simulink model "sim_all_2019b"  (R2019b)
settings: Solver=VariableStepAuto  StartTime=0.0  StopTime=2000  RelTol=1e-3
undefined symbols (not defined in the file or in its folder): a1, a2, alpha1, alpha2, cornerA, cornerB, cornerC, cornerD, ctrl_clockwise, ctrl_int_bound_or, ctrl_int_bound_pos, ctrl_k_or, ctrl_k_pos, ctrl_Ki_vel, ctrl_Kp_v_pos, ctrl_Kp_vel, ctrl_TAM, ctrl_Ts, ctrl_va_uncontrolled, ctrl_vel_uncontrolled, D, dead_zone_limit, depth, DiscIntNeverNeededParam, distanceFromWall, initInspectedSide, initPoint, mod_A, mod_Cd_F, mod_Cd_M, mod_eta_init, mod_g, mod_h0, mod_Ixx, mod_Iyy, mod_Izz, mod_Kp_dot, mod_lat0, mod_lon0, mod_m, mod_Mq_dot, mod_ni_init, mod_Nr_dot, mod_p1, mod_p2, mod_p3, mod_p4, mod_p5, mod_p6, mod_R, mod_Rm, mod_t1, mod_t2, mod_t3, mod_t4, mod_t5, mod_t6, mod_W, mod_Xu_dot, mod_Yv_dot ... (+53)
libraries: simulink x8, cstblocks x6, simulink_extras x1
(part 3 of 6)

== system sim_all_2019b/Mission_supervisor_v3/Mission_Supervisor/Orientazione in profondità ==
  Pos_s : Inport
  Orp_s : Inport  Port=2
  Punto_iniz_patt : Inport  Port=3
  error_flag : Inport  Port=4
  Action Port : ActionPort  ActionPortLabel=case [ 104 ]:
  Constant{,1..3,6} (5 alike) : Constant  Value=nan
  MATLAB Function : MATLAB Function  TreatAsAtomicUnit=on  SystemSampleTime=Ts_supervisor
  Mux : Mux  Inputs=6
  Mux1 : Mux  Inputs=3
  delta_current_or_prof : Outport
  delta_stato_or_prof : Outport  Port=2
  Outport : Outport  Port=3
  wires:
  MATLAB Function/1(delta_current_or_prof) -> delta_current_or_prof/1
  MATLAB Function/2(delta_stato_or_prof) -> delta_stato_or_prof/1
  MATLAB Function/3(Pos_d) -> Mux/1
  Mux/1 -> Outport/1
  Constant1/1 -> Mux/3
  MATLAB Function/4(Dpp_d) -> Mux/4
  MATLAB Function/5(Orp_d) -> Mux/6
  Constant/1 -> Mux1/1
  Constant2/1 -> Mux1/2
  Constant6/1 -> Mux1/3
  Mux1/1 -> Mux/2
  Constant3/1 -> Mux/5
  Pos_s/1 -> MATLAB Function/1(Pos_s)
  Orp_s/1 -> MATLAB Function/2(Orp_s)
  Punto_iniz_patt/1 -> MATLAB Function/3(punto_iniz_patt)
  error_flag/1 -> MATLAB Function/4(error_flag)

== system sim_all_2019b/Mission_supervisor_v3/Mission_Supervisor/Orientazione in superficie ==
  Or_in : Inport
  error_flag : Inport  Port=2
  punto_iniz_patt : Inport  Port=3
  Pos_s : Inport  Port=4
  Or_s : Inport  Port=5
  Action Port : ActionPort  ActionPortLabel=case [ 302 ]:
  Constant{1..2,4..5} (4 alike) : Constant  Value=nan
  MATLAB Function : MATLAB Function  TreatAsAtomicUnit=on  SystemSampleTime=Ts_supervisor
  Mux : Mux  Inputs=6
  delta_current_or_sup : Outport
  delta_stato_or_sup : Outport  Port=2
  Outport : Outport  Port=3
  wires:
  Mux/1 -> Outport/1
  Constant1/1 -> Mux/3
  Constant4/1 -> Mux/5
  Or_in/1 -> MATLAB Function/1(Or_in)
  error_flag/1 -> MATLAB Function/2(error_flag)
  punto_iniz_patt/1 -> MATLAB Function/3(punto_iniz_patt)
  MATLAB Function/1(delta_current_or_sup) -> delta_current_or_sup/1
  MATLAB Function/2(delta_stato_or_sup) -> delta_stato_or_sup/1
  MATLAB Function/4(Or_d) -> Mux/2
  MATLAB Function/3(Pos_d) -> Mux/1
  Constant2/1 -> Mux/4
  Constant5/1 -> Mux/6
  Pos_s/1 -> MATLAB Function/4(Pos_s)
  Or_s/1 -> MATLAB Function/5(Or_s)

== system sim_all_2019b/Mission_supervisor_v3/Mission_Supervisor/Pattugliamento ==
  parete : Inport
  contatore : Inport  Port=2
  Pos_s : Inport  Port=3
  Dpp_s : Inport  Port=4
  Dps_s : Inport  Port=5
  Orp_s : Inport  Port=6
  Vel_s : Inport  Port=7
  error_flag : Inport  Port=8
  giro : Inport  Port=9
  Action Port : ActionPort  ActionPortLabel=case [ 201 ]:
  Constant{,1..2,6} (4 alike) : Constant  Value=nan
  MATLAB Function : MATLAB Function  TreatAsAtomicUnit=on  SystemSampleTime=Ts_supervisor
  Mux : Mux  Inputs=6
  Mux1 : Mux  Inputs=3
  delta_current_patt : Outport
  delta_stato_patt : Outport  Port=2
  Outport : Outport  Port=3
  wires:
  MATLAB Function/1(delta_current_patt) -> delta_current_patt/1
  MATLAB Function/2(delta_stato_patt) -> delta_stato_patt/1
  parete/1 -> MATLAB Function/1(parete)
  contatore/1 -> MATLAB Function/2(contatore)
  MATLAB Function/3(Pos_d) -> Mux/1
  Mux/1 -> Outport/1
  Mux1/1 -> Mux/2
  MATLAB Function/4(Vel_d) -> Mux/3
  MATLAB Function/5(Dpp_d) -> Mux/4
  Constant/1 -> Mux1/1
  Constant2/1 -> Mux1/2
  Constant6/1 -> Mux1/3
  Pos_s/1 -> MATLAB Function/3(Pos_s)
  Dpp_s/1 -> MATLAB Function/4(Dpp_s)
  Dps_s/1 -> MATLAB Function/5(Dps_s)
  Vel_s/1 -> MATLAB Function/7(Vel_s)
  Orp_s/1 -> MATLAB Function/6(Orp_s)
  error_flag/1 -> MATLAB Function/8(error_flag)
  giro/1 -> MATLAB Function/9(giro)
  Constant1/1 -> Mux/5
  MATLAB Function/6(Orp_d) -> Mux/6

== system sim_all_2019b/Mission_supervisor_v3/Mission_Supervisor/Posizionamento ==
  Pos_s : Inport
  Or_s : Inport  Port=2
  punto iniziale : Inport  Port=3
  Or_in : Inport  Port=4
  error_flag : Inport  Port=5
  Action Port : ActionPort  ActionPortLabel=case [ 102 ]:
  Constant{,1..3} (4 alike) : Constant  Value=nan
  MATLAB Function : MATLAB Function  TreatAsAtomicUnit=on  SystemSampleTime=Ts_supervisor
  Mux : Mux  Inputs=6
  delta_current_posiz : Outport
  delta_stato_posiz : Outport  Port=2
  Outport : Outport  Port=3
  wires:
  MATLAB Function/1(delta_current_posiz) -> delta_current_posiz/1
  MATLAB Function/2(delta_stato_posiz) -> delta_stato_posiz/1
  MATLAB Function/3(Pos_d) -> Mux/1
  MATLAB Function/4(Or_d) -> Mux/2
  Mux/1 -> Outport/1
  Constant/1 -> Mux/3
  Constant1/1 -> Mux/6
  Constant2/1 -> Mux/5
  Pos_s/1 -> MATLAB Function/1(Pos_s)
  punto iniziale/1 -> MATLAB Function/3(punto_iniziale)
  Or_in/1 -> MATLAB Function/4(Or_in)
  Or_s/1 -> MATLAB Function/2(Or_s)
  error_flag/1 -> MATLAB Function/5(error_flag)
  Constant3/1 -> Mux/4

== system sim_all_2019b/Mission_supervisor_v3/Mission_Supervisor/Rientro ==
  Pos_s : Inport
  Or_in : Inport  Port=2
  error_flag : Inport  Port=3
  Dps_s : Inport  Port=4
  Dpp_s : Inport  Port=5
  Or_s : Inport  Port=6
  Action Port : ActionPort  ActionPortLabel=case [ 303 ]:
  Constant{1..4} (4 alike) : Constant  Value=nan
  MATLAB Function : MATLAB Function  TreatAsAtomicUnit=on  SystemSampleTime=Ts_supervisor
  Mux : Mux  Inputs=6
  delta_current_rient : Outport
  delta_stato_rient : Outport  Port=2
  Outport : Outport  Port=3
  wires:
  MATLAB Function/1(delta_current_rient) -> delta_current_rient/1
  MATLAB Function/2(delta_stato_rient) -> delta_stato_rient/1
  MATLAB Function/3(Pos_d) -> Mux/1
  Mux/1 -> Outport/1
  Constant1/1 -> Mux/3
  Constant2/1 -> Mux/4
  Constant3/1 -> Mux/5
  Constant4/1 -> Mux/6
  Pos_s/1 -> MATLAB Function/1(Pos_s)
  MATLAB Function/4(Or_d) -> Mux/2
  Or_in/1 -> MATLAB Function/2(Or_in)
  error_flag/1 -> MATLAB Function/3(error_flag)
  Dps_s/1 -> MATLAB Function/4(Dps_s)
  Dpp_s/1 -> MATLAB Function/5(Dpp_s)
  Or_s/1 -> MATLAB Function/6(Or_s)

== system sim_all_2019b/Mission_supervisor_v3/Mission_Supervisor/Risalita ==
  delta_SOS : Inport
  Pos_s : Inport  Port=2
  Dpp_s : Inport  Port=3
  Orp_s : Inport  Port=4
  Dps_s : Inport  Port=5
  Dps_fin : Inport  Port=6
  error_flag : Inport  Port=7
  SOS_205 : Inport  Port=8
  Action Port : ActionPort  ActionPortLabel=case [ 301 ]:
  Constant{,1,3,6} (4 alike) : Constant  Value=nan
  MATLAB Function : MATLAB Function  TreatAsAtomicUnit=on  SystemSampleTime=Ts_supervisor
  Mux : Mux  Inputs=6
  Mux1 : Mux  Inputs=3
  delta_current_ris : Outport
  delta_stato_ris : Outport  Port=2
  Outport : Outport  Port=3
  wires:
  MATLAB Function/1(delta_current_ris) -> delta_current_ris/1
  MATLAB Function/2(delta_stato_ris) -> delta_stato_ris/1
  MATLAB Function/3(Pos_d) -> Mux/1
  Mux/1 -> Outport/1
  Mux1/1 -> Mux/2
  Constant1/1 -> Mux/3
  MATLAB Function/4(Dpp_d) -> Mux/4
  Constant/1 -> Mux1/1
  Constant3/1 -> Mux1/2
  Constant6/1 -> Mux1/3
  MATLAB Function/5(Dps_d) -> Mux/5
  Pos_s/1 -> MATLAB Function/2(Pos_s)
  Dpp_s/1 -> MATLAB Function/3(Dpp_s)
  MATLAB Function/6(Orp_d) -> Mux/6
  delta_SOS/1 -> MATLAB Function/1(delta_SOS)
  Orp_s/1 -> MATLAB Function/4(Orp_s)
  Dps_s/1 -> MATLAB Function/5(Dps_s)
  Dps_fin/1 -> MATLAB Function/6(Dps_fin)
  error_flag/1 -> MATLAB Function/7(error_flag)
  SOS_205/1 -> MATLAB Function/8(SOS_205)

== system sim_all_2019b/Model/Vehicle Model/P1 ==
  note: n is the rotational speed of the thruster
      | V is the speed component of the water along the thruster axis
      |
      | n is saturated according to data
      | a dead zone is considered according to data
      | the thruster is characterised by 1st order dynamics (tau = 0.2s)
  n1 [rad/s] : Inport
  V1 [m/s] : Inport  Port=2
  Dead Zone : DeadZone  LowerValue=-dead_zone_limit  UpperValue=dead_zone_limit  SaturateOnIntegerOverflow=on
  Propeller1 : MATLAB Function  TreatAsAtomicUnit=on
  Saturation : Saturate  UpperLimit=n_max  LowerLimit=-n_max
  Transfer Fcn : TransferFcn  Denominator=[0.2 1]
  T1 : Outport
  wires:
  V1 [m/s]/1 -> Propeller1/2(V1)
  Saturation/1 -> Propeller1/1(n1)
  Transfer Fcn/1 -> Saturation/1
  Dead Zone/1 -> Transfer Fcn/1
  n1 [rad/s]/1 -> Dead Zone/1
  Propeller1/1(T1) -> T1/1

== system sim_all_2019b/Model/Vehicle Model/P2 ==
  note: n is the rotational speed of the thruster
      | V is the speed component of the water along the thruster axis
      |
      | n is saturated according to data
      | a dead zone is considered according to data
      | the thruster is characterised by 1st order dynamics (tau = 0.2s)
  n2 [rad/s] : Inport
  V2 [m/s] : Inport  Port=2
  Dead Zone : DeadZone  LowerValue=-dead_zone_limit  UpperValue=dead_zone_limit  SaturateOnIntegerOverflow=on
  Propeller2 : MATLAB Function  TreatAsAtomicUnit=on
  Saturation : Saturate  UpperLimit=n_max  LowerLimit=-n_max
  Transfer Fcn : TransferFcn  Denominator=[0.2 1]
  T2 : Outport
  wires:
  V2 [m/s]/1 -> Propeller2/2(V2)
  Saturation/1 -> Propeller2/1(n2)
  Transfer Fcn/1 -> Saturation/1
  Dead Zone/1 -> Transfer Fcn/1
  n2 [rad/s]/1 -> Dead Zone/1
  Propeller2/1(T2) -> T2/1

== system sim_all_2019b/Model/Vehicle Model/P3 ==
  note: n is the rotational speed of the thruster
      | V is the speed component of the water along the thruster axis
      |
      | n is saturated according to data
      | a dead zone is considered according to data
      | the thruster is characterised by 1st order dynamics (tau = 0.2s)
  n3 [rad/s] : Inport
  V3 [m/s] : Inport  Port=2
  Dead Zone : DeadZone  LowerValue=-dead_zone_limit  UpperValue=dead_zone_limit  SaturateOnIntegerOverflow=on
  Propeller3 : MATLAB Function  TreatAsAtomicUnit=on
  Saturation : Saturate  UpperLimit=n_max  LowerLimit=-n_max
  Transfer Fcn : TransferFcn  Denominator=[0.2 1]
  T3 : Outport
  wires:
  V3 [m/s]/1 -> Propeller3/2(V3)
  Saturation/1 -> Propeller3/1(n3)
  Transfer Fcn/1 -> Saturation/1
  Dead Zone/1 -> Transfer Fcn/1
  n3 [rad/s]/1 -> Dead Zone/1
  Propeller3/1(T3) -> T3/1

== system sim_all_2019b/Model/Vehicle Model/P4 ==
  note: n is the rotational speed of the thruster
      | V is the speed component of the water along the thruster axis
      |
      | n is saturated according to data
      | a dead zone is considered according to data
      | the thruster is characterised by 1st order dynamics (tau = 0.2s)
  n4 [rad/s] : Inport
  V4 [m/s] : Inport  Port=2
  Dead Zone : DeadZone  LowerValue=-dead_zone_limit  UpperValue=dead_zone_limit  SaturateOnIntegerOverflow=on
  Propeller4 : MATLAB Function  TreatAsAtomicUnit=on
  Saturation : Saturate  UpperLimit=n_max  LowerLimit=-n_max
  Transfer Fcn : TransferFcn  Denominator=[0.2 1]
  T4 : Outport
  wires:
  V4 [m/s]/1 -> Propeller4/2(V4)
  Saturation/1 -> Propeller4/1(n4)
  Transfer Fcn/1 -> Saturation/1
  Dead Zone/1 -> Transfer Fcn/1
  n4 [rad/s]/1 -> Dead Zone/1
  Propeller4/1(T4) -> T4/1

== system sim_all_2019b/Model/Vehicle Model/P5 ==
  note: n is the rotational speed of the thruster
      | V is the speed component of the water along the thruster axis
      |
      | n is saturated according to data
      | a dead zone is considered according to data
      | the thruster is characterised by 1st order dynamics (tau = 0.2s)
  n5 [rad/s] : Inport
  V5 [m/s] : Inport  Port=2
  Dead Zone : DeadZone  LowerValue=-dead_zone_limit  UpperValue=dead_zone_limit  SaturateOnIntegerOverflow=on
  Propeller5 : MATLAB Function  TreatAsAtomicUnit=on
  Saturation : Saturate  UpperLimit=n_max  LowerLimit=-n_max
  Transfer Fcn : TransferFcn  Denominator=[0.2 1]
  T5 : Outport
  wires:
  V5 [m/s]/1 -> Propeller5/2(V5)
  Saturation/1 -> Propeller5/1(n5)
  Transfer Fcn/1 -> Saturation/1
  Dead Zone/1 -> Transfer Fcn/1
  n5 [rad/s]/1 -> Dead Zone/1
  Propeller5/1(T5) -> T5/1

== system sim_all_2019b/Model/Vehicle Model/P6 ==
  note: n is the rotational speed of the thruster
      | V is the speed component of the water along the thruster axis
      |
      | n is saturated according to data
      | a dead zone is considered according to data
      | the thruster is characterised by 1st order dynamics (tau = 0.2s)
  n6 [rad/s] : Inport
  V6 [m/s] : Inport  Port=2
  Dead Zone : DeadZone  LowerValue=-dead_zone_limit  UpperValue=dead_zone_limit  SaturateOnIntegerOverflow=on
  Propeller6 : MATLAB Function  TreatAsAtomicUnit=on
  Saturation : Saturate  UpperLimit=n_max  LowerLimit=-n_max
  Transfer Fcn : TransferFcn  Denominator=[0.2 1]
  T6 : Outport
  wires:
  V6 [m/s]/1 -> Propeller6/2(V6)
  Saturation/1 -> Propeller6/1(n6)
  Transfer Fcn/1 -> Saturation/1
  Dead Zone/1 -> Transfer Fcn/1
  n6 [rad/s]/1 -> Dead Zone/1
  Propeller6/1(T6) -> T6/1

== system sim_all_2019b/Navigation/Extended Kalman Filter/AHRS__check ==
  AHRS_new : Inport
  MATLAB Function4 : MATLAB Function  TreatAsAtomicUnit=on
  Memory4 : Memory
  flag_AHRS : Outport
  AHRS_now : Outport  Port=2
  wires:
  AHRS_new/1 -> MATLAB Function4/1(AHRS_new)
  Memory4/1 -> MATLAB Function4/2(AHRS_old)
  MATLAB Function4/1(flag_AHRS) -> flag_AHRS/1
  MATLAB Function4/2(AHRS_now) -> Memory4/1, AHRS_now/1

== system sim_all_2019b/Navigation/Extended Kalman Filter/CORREZIONE ==
  x_k|k-1 : Inport
  P_k|k-1 : Inport  Port=2
  e : Inport  Port=3
  H : Inport  Port=4
  R : Inport  Port=5
  nav_flag_init : Inport  Port=6
  MATLAB Function : MATLAB Function  TreatAsAtomicUnit=on  SystemSampleTime=nav_DT
  x_k|k : Outport
  P_k|k : Outport  Port=2
  wires:
  x_k|k-1/1 -> MATLAB Function/1(x_k_k_1)
  P_k|k-1/1 -> MATLAB Function/2(P_k_k_1)
  e/1 -> MATLAB Function/3(e)
  H/1 -> MATLAB Function/4(H)
  MATLAB Function/1(x_k) -> x_k|k/1
  MATLAB Function/2(P_k) -> P_k|k/1
  nav_flag_init/1 -> MATLAB Function/6(nav_flag_init)
  R/1 -> MATLAB Function/5(R_k)

== system sim_all_2019b/Navigation/Extended Kalman Filter/DVL_check ==
  DVL_new : Inport
  MATLAB Function4 : MATLAB Function  TreatAsAtomicUnit=on
  Memory4 : Memory
  flag_DVL : Outport
  DVL_now : Outport  Port=2
  wires:
  DVL_new/1 -> MATLAB Function4/1(DVL_new)
  Memory4/1 -> MATLAB Function4/2(DVL_old)
  MATLAB Function4/1(flag_DVL) -> flag_DVL/1
  MATLAB Function4/2(DVL_now) -> Memory4/1, DVL_now/1

== system sim_all_2019b/Navigation/Extended Kalman Filter/MISURA VIRTUALE ==
  x_k|k-1 : Inport
  flag_vect : Inport  Port=2
  mis_vect : Inport  Port=3
  J : Inport  Port=4
  MATLAB Function : MATLAB Function  TreatAsAtomicUnit=on  SystemSampleTime=nav_DT
  e : Outport
  H : Outport  Port=2
  wires:
  x_k|k-1/1 -> MATLAB Function/1(x_k_k_1)
  mis_vect/1 -> MATLAB Function/3(mis_vect)
  flag_vect/1 -> MATLAB Function/2(flag_vect)
  MATLAB Function/1(e) -> e/1
  MATLAB Function/2(H) -> H/1
  J/1 -> MATLAB Function/4(J)

== system sim_all_2019b/Navigation/Extended Kalman Filter/PREDIZIONE ==
  x0 : Inport
  P0 : Inport  Port=2
  x_k-1|k-1 : Inport  Port=3
  u_k-1 : Inport  Port=4
  P_k-1|k-1 : Inport  Port=5
  J : Inport  Port=6
  L : Inport  Port=7
  Q_k-1 : Inport  Port=8
  nav_flag_init : Inport  Port=9
  Passo di Predizione : MATLAB Function  TreatAsAtomicUnit=on  SystemSampleTime=nav_DT
  x_k|k-1 : Outport
  P_k|k-1 : Outport  Port=2
  flag_init : Outport  Port=3
  wires:
  Passo di Predizione/1(x_k) -> x_k|k-1/1
  Passo di Predizione/2(P_k) -> P_k|k-1/1
  u_k-1/1 -> Passo di Predizione/4(u_k_1)
  x_k-1|k-1/1 -> Passo di Predizione/3(x_k_1)
  P_k-1|k-1/1 -> Passo di Predizione/5(P_k_1)
  J/1 -> Passo di Predizione/6(J)
  Q_k-1/1 -> Passo di Predizione/8(Q_k_1)
  P0/1 -> Passo di Predizione/2(P0)
  x0/1 -> Passo di Predizione/1(x0)
  L/1 -> Passo di Predizione/7(L)
  nav_flag_init/1 -> Passo di Predizione/9("nav_flag_init ")
  Passo di Predizione/3(nav_flag_init) -> flag_init/1

== system sim_all_2019b/Navigation/Extended Kalman Filter/Q_error ==
  flag_AHRS : Inport
  flag_DVL : Inport  Port=2
  Q : Inport  Port=3
  MATLAB Function4 : MATLAB Function  TreatAsAtomicUnit=on
  Memory : Memory
  Q_k : Outport
  wires:
  MATLAB Function4/1(Q_k) -> Q_k/1, Memory/1
  flag_AHRS/1 -> MATLAB Function4/3(flag_AHRS)
  flag_DVL/1 -> MATLAB Function4/4(flag_DVL)
  Memory/1 -> MATLAB Function4/2(Q_k_1)
  Q/1 -> MATLAB Function4/1(Q)

== system sim_all_2019b/Sensors/BLOCCO GYRO1/Subsystem ==
  t : Inport  SampleTime=sens_Sample_time_GYRO
  GEOD to NED : MATLAB Function  TreatAsAtomicUnit=on
  Bias_G : Outport
  wires:
  t/1 -> GEOD to NED/1(t)
  GEOD to NED/1(Bias_G) -> Bias_G/1

== matlab function sim_all_2019b/Mission_supervisor_v3/Mission_Supervisor/MATLAB Function1 ==
  data: punto_iniz_patt output size=3; initInspectedSide parameter; distanceFromWall parameter; initPoint parameter; Or_in output; dps_fin output; cornerA parameter; cornerB parameter; cornerC parameter; cornerD parameter; relativeDirection parameter; alfa output
function [punto_iniz_patt, Or_in, dps_fin, alfa] = ambiente(initInspectedSide,distanceFromWall,initPoint,cornerA, cornerB, cornerC, cornerD, relativeDirection)
 
    %% Unità di misura 
    
    % punto_iniz_patt, initPoint, cornerA, cornerB, cornerC, cornerD        [deg, deg, m]
    % Or_in                                                                 [rad, rad, rad]
    % dps_fin,distanceFromWall                                              [m]
    % alfa                                                                  [rad]
    % relativeDirection                                                     [deg]

    %% Inizializzazione variabili
    
    % Valori dati da file relativi agli angoli del bacino
    iP = initPoint;
    A = cornerA;
    B = cornerB;
    C = cornerC;
    D = cornerD;

    coder.extrinsic('evalin', 'wgs84Ellipsoid', 'geodetic2ned');
    coder.extrinsic('evalin', 'wgs84Ellipsoid', 'ned2geodetic');

    % Inizializzazione di alcune variabili
    xA = 0; yA = 0; zA = 0; xB = 0; yB = 0; zB = 0; xC = 0; yC = 0; zC = 0; 
    xD = 0; yD = 0; zD = 0; xiP = 0; yiP = 0; ziP = 0;
    xpipAB = 0; ypipAB = 0; zpipAB = 0; xpipBC = 0; ypipBC = 0; zpipBC = 0; 
    xpipCD = 0; ypipCD = 0; zpipCD = 0; xpipDA = 0; ypipDA = 0; zpipDA = 0;
    depth_in = initPoint(3);
    Or_in = [0; 0; 0];
    
    % Conversione da Geodetic a NED delle posizioni degli angoli e del punto iniziale
    wgs84 = wgs84Ellipsoid; % Per il corretto funzionamento e' necessario installare un 
                            % pacchetto aggiuntivo in Matlab qualora non fosse presente
    [xA, yA, zA] = geodetic2ned(A(1), A(2), 0, C(1), C(2), 0, wgs84);
    [xB, yB, zB] = geodetic2ned(B(1), B(2), 0, C(1), C(2), 0, wgs84);
    [xC, yC, zC] = geodetic2ned(C(1), C(2), 0, C(1), C(2), 0, wgs84);
    [xD, yD, zD] = geodetic2ned(D(1), D(2), 0, C(1), C(2), 0, wgs84);
    [xiP, yiP, ziP] = geodetic2ned(iP(1), iP(2), 0, C(1), C(2), 0, wgs84);
    inizio = [xiP; yiP; depth_in];

    % Punti centrali delle pareti
    pcAB = [(xB + xA)/2; (yB + yA)/2; depth_in];
    pcBC = [(xB + xC)/2; (yB + yC)/2; depth_in];   
    pcCD = [(xC + xD)/2;(yC + yD)/2; depth_in];
    pcDA = [(xD + xA)/2; (yD + yA)/2; depth_in];

    % Lunghezze delle pareti
    AB = sqrt((xA - xB)^2 + (yA - yB)^2); 
    BC = sqrt((xB - xC)^2 + (yB - yC)^2); 
    CD = sqrt((xC - xD)^2 + (yC - yD)^2); 
    DA = sqrt((xD - xA)^2 + (yD - yA)^2); 
    
    dW = distanceFromWall;

    %% Calcolo punto di inizio pattugliamento a meta' parete

    % Calcolo degli angoli relativi tra le pareti 
    thetaBC = acos(yB/BC);          
    thetaCD = acos(yD/CD);
    gammaAB = acos((yB - yA)/AB);
    thetaAB = pi - gammaAB;
    gammaDA = acos((yA - yD)/DA);

    % Punti di inizio pattugliamento a seconda di quale parete è scelta come
    % parete iniziale
    
    dbpc = sqrt((pcAB(1) - xB)^2 + (pcAB(2) - yB)^2);
    hpb = sqrt(dbpc^2 + dW^2);
    alfa1 = - acos(dbpc/hpb);
    gammaab = pi - (gammaAB + alfa1);
    pcab1 = [hpb * sin(gammaab), hpb * cos(gammaab)];
    pipAB = [xB + pcab1(1); yB + pcab1(2); depth_in];

    dcpc = sqrt(pcBC(1)^2 + pcBC(2)^2);
    hpc = sqrt(dcpc^2 + dW^2);
    alfabc = acos(dcpc/hpc);
    gammaBC = thetaBC + alfabc;
    pipBC = [hpc * sin(gammaBC); hpc * cos(gammaBC); depth_in];

    dcdpc = sqrt(pcCD(1)^2 + pcCD(2)^2);
    hpcd = sqrt(dcdpc^2 + dW^2);
    alfacd = acos(dcdpc/hpcd);
    gammaCD = thetaCD - alfacd;
    pipCD = [hpcd * sin(gammaCD); hpcd * cos(gammaCD); depth_in];

    dapc = sqrt((pcDA(1) - xA)^2 + (pcDA(2) - yA)^2);
    hpda = sqrt(dapc^2 + dW^2);
    alfada = acos(dapc/hpda);
    gammada = pi + (gammaDA + alfada);
    pcda1 = [hpda * sin(gammada), hpda * cos(gammada)];
    pipDA = [xA + pcda1(1); yA + pcda1(2); depth_in];
    
    % Si convertono i punti "pip" da NED a Geodetic 
    [xpipAB, ypipAB, zpipAB] = ned2geodetic(pipAB(1), pipAB(2), pipAB(3), C(1), C(2), 0, wgs84);
    [xpipBC, ypipBC, zpipBC] = ned2geodetic(pipBC(1), pipBC(2), pipBC(3), C(1), C(2), 0, wgs84);
    [xpipCD, ypipCD, zpipCD] = ned2geodetic(pipCD(1), pipCD(2), pipCD(3), C(1), C(2), 0, wgs84);
    [xpipDA, ypipDA, zpipDA] = ned2geodetic(pipDA(1), pipDA(2), pipDA(3), C(1), C(2), 0, wgs84);

    pipAB_geodetic = [xpipAB; ypipAB; depth_in];
    pipBC_geodetic = [xpipBC; ypipBC; depth_in];
    pipCD_geodetic = [xpipCD; ypipCD; depth_in];
    pipDA_geodetic = [xpipDA; ypipDA; depth_in];

    %% Calcolo angolo di orientazione iniziale in direzione del punto di inizio  pattugliamento (rispetto al nord)

    % Versore orinetato verso il nord n = [1, 0, 0];
    
    % Vettori che vanno dal punto di partenza al punto di inizio pattugliamento
    
    iAB = pipAB - inizio;
    iBC = pipBC - inizio;
    iCD = pipCD - inizio;
    iDA = pipDA - inizio;

    % Angoli tra direzione Nord e il vettore che porta verso il punto di inizio pattugliamento. 
    % Sono gli angoli di orientazione iniziale desiderata. 
    theta1 = atan2d(iAB(2),iAB(1));
    theta2 = atan2d(iBC(2),iBC(1));
    theta3 = atan2d(iCD(2),iCD(1));
    theta4 = atan2d(iDA(2),iDA(1));
    
    % Si raccoglie in un vettore
    theta = [deg2rad(theta1), deg2rad(theta2), deg2rad(theta3), deg2rad(theta4)];

    %% Si calcolano gli angoli interni dei vertici
    
    alfaC = thetaCD - thetaBC;
    alfaB = pi - (thetaAB-thetaBC);
    alfaA = thetaAB - gammaDA;
    alfaD = 2*pi - alfaA - alfaB - alfaC;
    alfa = [alfaA; alfaB; alfaC; alfaD];    %Utilizzati poi in fase di manovra

    %% Calcolo distanza dalla parete successiva a partire da meta'  parete

    % Sono le distanze da metà parete alla parete successiva
    dABpc = sqrt((pcAB(1) - xB)^2 + (pcAB(2) - yB)^2);
    dBCpc = sqrt(pcBC(1)^2 + pcBC(2)^2);
    dCDpc = sqrt(pcCD(1)^2 + pcCD(2)^2);
    dDApc = sqrt((pcDA(1) - xA)^2 + (pcDA(2) - yA)^2);


    %% Scelta delle condizioni

    % In base al valore di parete iniziale si assegnano i giusti valori per i 
    % riferimenti da utilizzare nei vari stati
    
    if initInspectedSide == 1

        punto_iniz_patt = pipAB_geodetic;
        Or_in = [0; 0; theta(1)];
        dps_fin = dABpc;

    elseif initInspectedSide == 2

        punto_iniz_patt = pipBC_geodetic;
        Or_in = [0; 0; theta(2)];
        dps_fin = dBCpc;

    elseif initInspectedSide == 3

        punto_iniz_patt = pipCD_geodetic;
        Or_in = [0; 0; theta(3)];
        dps_fin = dCDpc;

    else

        punto_iniz_patt = pipDA_geodetic;
        Or_in = [0; 0; theta(4)];
        dps_fin = dDApc;

    end
                                                                            %****TEST*****%
                                                                            %Or_in = [1; 1; 1];

end

== matlab function sim_all_2019b/Controller_mk4_v3/C_pos/C_pos_Y ==
  data: err_int output; pos input; vel output; k input; ctrl_vel_uncontrolled parameter; ctrl_int_bound_pos parameter
%% Azione proporzionale
function [err_int, vel] = fcn(pos, k, ctrl_vel_uncontrolled, ctrl_int_bound_pos)
    v = 0;
    err_int = 0;
    vel_des = ctrl_vel_uncontrolled;    % velocità impostata se 'lontani'
    brake_dist = 1/k*vel_des;           % distanza di frenata
    if pos >= brake_dist                % se ho spazio per frenare mantengo la velocità
        v = vel_des;
    end
    if pos <= -brake_dist               % lontani in direzione negativa
        v = -vel_des;
    end
    if  abs(pos) < brake_dist           % se è vicino il proporzionale gestisce la frenata
        v = k*pos;
    end
    vel = v;
    if abs(pos) < ctrl_int_bound_pos    % per il regime può essere utile una azione integrale
        err_int = pos;                  % err_int va ad un integratore
    end

== matlab function sim_all_2019b/Mission_supervisor_v3/Mission_Supervisor/Inizio/MATLAB Function ==
  data: current_state output; parete_attuale output; stato_interno output; Pos_d output size=3; Pos_s input; error_flag input; attesa input; initInspectedSide parameter; initPoint parameter; timer parameter; SOS parameter
function [current_state, parete_attuale, stato_interno, Pos_d] =  Inizio(Pos_s, error_flag, attesa, initInspectedSide, initPoint, timer, SOS)
    
    disp("Inizio");
    
    %% Unita' di misura
    
    % Pos_d, Pos_s, initPoint                                                [deg, deg, m]
    % attesa, timer                                                          [s]
    
    %% Inizializzazione variabili
    
    % Mantenimento di stato_interno al valore
    % desiderato durante la permanenza del sistema nello stato corrente.
    stato_interno = 100;

    % Se non si ricevono dati dal GPS per un tempo superiore ad una soglia
    % massima di attesa, la missione viene interrotta poiché non è
    % possibile localizzarsi nel bacino
    if ((isnan(Pos_s(1)) || isnan(Pos_s(2))) && (attesa > timer))
        SOS = 1;
        disp("EMERGENZA: mancata ricezione dati da GPS");
    end
    
    %% Preparazione dei riferimenti 
    
        % Parete di inizio pattugliamento
        parete_attuale = initInspectedSide;
        
        % Posizione di inizio missione
        Pos_d = initPoint; 
        
        
    %% Transizione di stato effettiva
    
        % Quando i riferimenti sono correttamente settati
        % viene comunicato agli altri moduli il passaggio di stato
        current_state = 100;  
        
    %% Decisione dello stato successivo
    
     if error_flag == 1
        disp("EMERGENZA: errore segnalato dagli altri sottosistemi");
        SOS = 1;
     end
    
    % Si verifica lo stato di emergenza e la ricezione di misure dal GPS
    if (SOS == 0 && ((isnan(Pos_s(1)) == false && isnan(Pos_s(2)) == false))) 
        
        stato_interno = 101;   % Si passa allo stato successivo
    else
        if SOS == 1
           
            stato_interno = 304; % Politica di emergenza: si passa in fine missione   
        end
    end

end

== matlab function sim_all_2019b/Mission_supervisor_v3/Mission_Supervisor/MATLAB Function ==
  data: parete_iniziale input; verso input; parete output; contatore input; initInspectedSide parameter; current_state input; giro output
function [parete, giro] = aggiorna_parete(parete_iniziale, verso, contatore, initInspectedSide,current_state)
   
 %% Corpo funzione 
    
    % A seconda del senso di pattugliamento si ha l'aggiornamento del valore
    % di parete attuale. 
    
    if(strcmp(verso,'clockwise') == 1)
        giro = 0;
        parete = mod((parete_iniziale + contatore),4);
        if(parete == 0)
            parete = 4;
        end
    else % 'counterclockwise'
        giro = 1;
        parete = parete_iniziale - contatore;
        if(parete <= 0)
            parete = parete+4;
        end
    end

    % Per stati precedenti al 201, si forza questa variabile a
    % mantenere il valore pari al valore iniziale. 
    if(current_state < 201)
        parete = initInspectedSide;
    end
    
end

== matlab function sim_all_2019b/Mission_supervisor_v3/Mission_Supervisor/Orientazione Iniziale/MATLAB Function ==
  data: delta_stato_or_iniz output; delta_current_or_iniz output; Pos_d output size=3; Pos_s input size=3; Or_s input size=3; Or_in input; initPoint parameter size=3; Or_d output size=3; error_flag input; soglia_or parameter; soglia_SOS_pos parameter; SOS parameter; soglia_SOS_or parameter
function [delta_stato_or_iniz, delta_current_or_iniz, Pos_d, Or_d] = Orientazione_iniziale(Pos_s, Or_s, Or_in, initPoint, error_flag, soglia_or, soglia_SOS_pos, SOS, soglia_SOS_or)

    disp("Orientazione iniziale");
    
    %% Unità di misura 
    
    % Pos_d, Pos_s, initPoint, soglia_SOS_pos                                [deg, deg, m]
    % Or_d, Or_s, Or_in, soglia_or, soglia_SOS_or                            [rad, rad, rad]
    
    %% Inizializzazione variabili
    
    % Mantenimento dello stato_interno al valore
    % desiderato durante la permanenza del sistema nello stato corrente.
    delta_stato_or_iniz = 0;
    
    % Variabile utilizzata per segnalare il momento in cui
    % effettuare la transizione di stato. 
    pronti = false;
    
    %% Preparazione dei riferimenti da fornire ai blocchi successivi
                
    % Posizione da mantenere
    Pos_d = initPoint; 
   
    % Orientazione desiderata per raggiungere
    % il punto di inizio pattugliamento
    Or_d = Or_in;
    
    % Quando i riferimenti sono correttamente settati
    % il passaggio di stato viene comunicato agli altri moduli
    delta_current_or_iniz = 101 - 100;
    
    
    %% Verifiche
    
    % Si verifica il mantenimento della posizione 
    % e la ricezione della stima di orientazione
    if (abs(Pos_s(1) - Pos_d(1)) > soglia_SOS_pos(1) || ...
        abs(Pos_s(2) - Pos_d(2)) > soglia_SOS_pos(2) || ...
        abs(Pos_s(3) - Pos_d(3)) > soglia_SOS_pos(3) || ...
        isnan(Or_s(1)) || isnan(Or_s(2)) || isnan(Or_s(3)) || ...
        abs(Or_s(1) - Or_d(1)) > soglia_SOS_or(1) || ...
        abs(Or_s(2) - Or_d(2)) > soglia_SOS_or(2))
    
        SOS = 1;
        disp("EMERGENZA:");
        
        if (abs(Pos_s(1) - Pos_d(1)) > soglia_SOS_pos(1))
            disp("Rilevato errore sulla posizione X");
        end
        if (abs(Pos_s(2) - Pos_d(2)) > soglia_SOS_pos(2))
            disp("Rilevato errore sulla posizione Y");
        end
        if (abs(Pos_s(3) - Pos_d(3)) > soglia_SOS_pos(3))
            disp("Rilevato errore sulla profondita Z");
        end
        if (isnan(Or_s(1)))
            disp("Mancata ricezione della prima componente di orientazione");
        end
        if (isnan(Or_s(2)))
            disp("Mancata ricezione della seconda componente di orientazione");
        end
        if (isnan(Or_s(3)))
            disp("Mancata ricezione della terza componente di orientazione");
        end
        if (abs(Or_s(1) - Or_d(1)) > soglia_SOS_or(1))
            disp("Rilevato errore sulla rotazione di roll");
        end
        if (abs(Or_s(2) - Or_d(2)) > soglia_SOS_or(2))
            disp("Rilevato errore sulla rotazione di pitch");
        end
    end

    if error_flag == 1
        disp("EMERGENZA: errore segnalato dagli altri sottosistemi");
        SOS = 1;
    end
    
    % Si verifica di aver raggiunto l'orientazione desiderata
    if (SOS == 0 && ...
        (abs(Or_s(3) - Or_d(3)) < soglia_or(3)))
    
        pronti = true;
        
    end
       
    %% Decisione dello stato successivo
    
    if pronti == true
        
        delta_stato_or_iniz = 102 - 101; % Transizione eseguita correttamente
    end
        
    if SOS == 1
            
            delta_stato_or_iniz = 304 - 101; % Transizione nello stato di emergenza
    end
    % Si rimane nello stato corrente

end

== matlab function sim_all_2019b/Mission_supervisor_v3/Mission_Supervisor/Immersione/MATLAB Function ==
  data: soglia_pos parameter; delta_current_immers output; delta_stato_immers output; Pos_d output size=3; Or_d output size=3; Pos_s input; depth parameter; punto_iniz_patt input; Or_in input; error_flag input; soglia_SOS_pos parameter; SOS parameter
function [delta_current_immers, delta_stato_immers, Pos_d, Or_d]=Immersione(soglia_pos, Pos_s, depth, punto_iniz_patt, Or_in, error_flag, soglia_SOS_pos, SOS)

    disp("Immersione");
    
    %% Unità di misura 
    
    % Pos_d, Pos_s, punto_iniz_patt, soglia_pos, soglia_SOS_pos            [deg, deg, m]
    % Or_d, Or_in                                                          [rad, rad, rad]
    % distanceFromWall, depth                                              [m]


    %% Inizializzazione variabili
    
    % Utilizzata durante la permanenza nello stato corrente
    delta_stato_immers = 0;
    
    pronti = false; 
    
    %% Preparazione dei riferimenti da fornire ai blocchi successivi
    
    % Posizione da raggiungere
    Pos_d = [punto_iniz_patt(1); punto_iniz_patt(2); depth];
                                                                            %*****TEST******%
                                                                            %Pos_d = [43; 11; 0];
    
    % Orientazione da mantenere
    Or_d = Or_in;
    
    % Transizione di stato effettiva
    delta_current_immers = 103 - 102;  
        
       
    %% Verifiche
    
    % Verifica della corretta posizione
    if (abs(Pos_s(1) - Pos_d(1)) > soglia_SOS_pos(1) || ...
        abs(Pos_s(2) - Pos_d(2)) > soglia_SOS_pos(2))
    
        SOS = 1;
        disp("EMERGENZA:"); 
        
        if (abs(Pos_s(1) - Pos_d(1)) > soglia_SOS_pos(1))
            disp("Rilevato errore sulla posizione X");
        end
        
        if (abs(Pos_s(2) - Pos_d(2)) > soglia_SOS_pos(2))
            disp("Rilevato errore sulla posizione Y");
        end

    end
    
    if error_flag == 1
        disp("EMERGENZA: errore segnalato dagli altri sottosistemi");
        SOS = 1;
    end
    
    % Si verifica di aver raggiunto la profondità desiderata 
    if (SOS == 0 && ...
        abs(Pos_s(3) - Pos_d(3)) < soglia_pos(3))
    
        pronti = true;
    end
    
    
    %% Decisione dello stato successivo
    
    if pronti == true
        
        delta_stato_immers = 104 - 103; % Transizione eseguita correttamente
    end 
    if SOS == 1
            
            delta_stato_immers = 301 - 103; % Transizione nello stato di emergenza
    end
    % Si rimane nello stato corrente

end

== matlab function sim_all_2019b/Mission_supervisor_v3/Mission_Supervisor/Orientazione in profondità/MATLAB Function ==
  data: delta_current_or_prof output; delta_stato_or_prof output; Pos_d output size=3; Dpp_d output; Orp_d output; Pos_s input; Orp_s input; relativeDirection parameter; depth parameter; punto_iniz_patt input; error_flag input; soglia_orp parameter; soglia_SOS_pos parameter; SOS parameter; distanceFromWall parameter
function [delta_current_or_prof, delta_stato_or_prof, Pos_d, Dpp_d, Orp_d] = Orientazione_profondita(Pos_s, Orp_s, relativeDirection, depth, punto_iniz_patt, error_flag, soglia_orp, soglia_SOS_pos, SOS, distanceFromWall)

    disp("Orientazione in profondita");
    
    %% Unità di misura 
    
    % Pos_d, Pos_s, punto_iniz_patt, soglia_SOS_pos                        [deg, deg, m]
    % Orp_d, Orp_s, soglia_orp                                             [rad]
    % relativeDirection                                                    [deg]
    % Dpp_d, depth, distanceFromWall                                       [m]

    %% Inizializzazione variabili
    
    % Utilizzata per la permanenza nello stato corrente
    delta_stato_or_prof = 0;
    
    pronti = false;

    %% Preparazione dei riferimenti da fornire ai blocchi successivi
                
    % Posizione da mantenere
    Pos_d = [punto_iniz_patt(1); punto_iniz_patt(2); depth];
                                                                            %*****TEST******%
                                                                            %Pos_d = [43; 11; 0];
    
  
    % Orientazione da raggiungere
    Orp_d = deg2rad(relativeDirection);
    
    % Distanza dalla parete da mantenere
    Dpp_d = distanceFromWall;
    
    
    % Transizione di stato effettiva
    delta_current_or_prof = 104 - 103; 
    
    
    %% Verifiche
    
    % Verifica della corretta posizione
    if (abs(Pos_s(1) - Pos_d(1)) > soglia_SOS_pos(1) || ...
        abs(Pos_s(2) - Pos_d(2)) > soglia_SOS_pos(2) || ...
        abs(Pos_s(3) - Pos_d(3)) > soglia_SOS_pos(3))
    
        SOS = 1;
        disp("EMERGENZA:");
        
        if (abs(Pos_s(1) - Pos_d(1)) > soglia_SOS_pos(1))
            disp("Rilevato errore sulla posizione X");
        end
        if (abs(Pos_s(2) - Pos_d(2)) > soglia_SOS_pos(2))
            disp("Rilevato errore sulla posizione Y");
        end
        if (abs(Pos_s(3) - Pos_d(3)) > soglia_SOS_pos(3))
            disp("Rilevato errore sulla profondita Z");
        end
        
    end
    
    if error_flag == 1
        disp("EMERGENZA: errore segnalato dagli altri sottosistemi");
        SOS = 1;
    end
     
    % Si verifica di aver raggiunto l'orientazione desiderata
    if (SOS == 0 && ...
        abs(Orp_s - Orp_d) < soglia_orp)
    
        pronti = true;
    end
    
    %% Decisione dello stato successivo
    
    if pronti == true
        
        delta_stato_or_prof = 201 - 104; % Transizione eseguita correttamente
    end
    if SOS == 1
            
            delta_stato_or_prof = 301 - 104; % Transizione nello stato di emergenza
    end
    
    % Si rimane nello stato corrente
    

end

== matlab function sim_all_2019b/Mission_supervisor_v3/Mission_Supervisor/Frenata pattugliamento/MATLAB Function ==
  data: delta_current_fren_patt output; delta_stato_fren_patt output; contatore input; Pos_d output size=3; Dpp_d output; Dps_d output; Orp_d output; Pos_s input; Dpp_s input; Dps_s input; Orp_s input; distanceFromWall parameter; relativeDirection parameter; depth parameter; error_flag input; soglia_SOS_orp parameter; soglia_SOS_pos parameter; soglia_SOS_parete parameter; SOS parameter; soglia_parete parameter
function [delta_current_fren_patt, delta_stato_fren_patt, Pos_d, Dpp_d, Dps_d, Orp_d] = Frenata_pattugliamento(contatore, Pos_s, Dpp_s, Dps_s, Orp_s, distanceFromWall, relativeDirection, depth, error_flag, soglia_SOS_orp, soglia_SOS_pos, soglia_SOS_parete, SOS,soglia_parete)

    disp("Frenata (durante il pattugliamento)");
    
    %% Unità di misura 
    
    % Pos_d, Pos_s, soglia_SOS_pos                                                                 [deg, deg, m]
    % Orp_d, Orp_s, soglia_SOS_orp                                                                 [rad]
    % relativeDirection                                                                            [deg]
    % Dpp_d, Dps_d, Dpp_s, Dps_s, distanceFromWall, depth, soglia_SOS_parete, soglia_parete        [m]

    %% Inizializzazione variabili
   
    % Utilizzata per permanere nello stato corrente
    delta_stato_fren_patt = contatore;
    
    pronti = false;
    
    %% Preparazione dei riferimenti da fornire ai blocchi successivi
    
    % Profondità da mantenere
    Pos_d = [nan; nan; depth];
                                                                            %*****TEST******%
                                                                            %Pos_d = [nan; nan; 0];
    
    % Distanza dalla parete da mantenere
    Dpp_d = distanceFromWall;
    Dps_d = distanceFromWall;
    
    % Orientazione da mantenere
    Orp_d = deg2rad(relativeDirection);
    
    % Transizione di stato effettiva
    delta_current_fren_patt = 202 - 201 + contatore;  
    
    
    %% Verifiche
    
    % Verifica sulla corretta orientazione, profondità e distanza dalla parete pattugliata
    if (abs(Orp_s - Orp_d) > soglia_SOS_orp || ...
        abs(Dpp_s - Dpp_d) > soglia_SOS_parete || ...
        abs(Pos_s(3) - Pos_d(3)) > soglia_SOS_pos(3))
    
        SOS = 1;
        disp("EMERGENZA:");
        
        if (abs(Orp_s - Orp_d) > soglia_SOS_orp)
            disp("Rilevato errore sull'orientazione relativa");
        end
        
        if (abs(Dpp_s - Dpp_d) > soglia_SOS_parete)
            disp("Rilevato errore sulla distanza da parete");
        end
        
        if (abs(Pos_s(3) - Pos_d(3)) > soglia_SOS_pos(3))
            disp("Rilevato errore sulla profondita Z");
        end
        
    end
    
    if error_flag == 1
        disp("EMERGENZA: errore segnalato dagli altri sottosistemi");
        SOS = 1;
    end
     
                                                                            %*****TEST******%
                                                                            %test=0;
                                                                            %Serve per testare di rimanere 
                                                                            %in attesa in questo stato
                                                                            % if(contatore>2)
                                                                            %    test=100;
                                                                            % else
                                                                            %    test=0;
                                                                            % end

    % Si verifica di aver raggiunto la posizione desiderata in termini di 
    % distanza dalla parete successiva
    if (SOS == 0 && ...
        abs(Dps_s - Dps_d) < soglia_parete)
    
        pronti = true;
        
    end

    %% Decisione dello stato successivo
    
    if pronti == true
        
        delta_stato_fren_patt = 203 - 202 + contatore; % Transizione eseguita correttamente
    end
    if SOS == 1
            
            delta_stato_fren_patt = 301 - 202 + contatore; % Transizione nello stato di emergenza
    end
    % Si rimane nello stato corrente

end

== matlab function sim_all_2019b/Mission_supervisor_v3/Mission_Supervisor/Manovra/MATLAB Function ==
  data: delta_current_man output; delta_stato_man output; contatore output; contatore input; Pos_d output size=3; Dpp_d output; Dps_d output; Orp_d output; Pos_s input; Dpp_s input; Orp_s input; distanceFromWall parameter; relativeDirection parameter; depth parameter; error_flag input; soglia_orp parameter; soglia_SOS_parete parameter; soglia_SOS_pos parameter; SOS parameter; Dps_s input; alfa input; giro input; parete_attuale input
function [delta_current_man, delta_stato_man, contatore, Pos_d, Dpp_d, Dps_d, Orp_d] = Manovra(contatore, Pos_s, Dpp_s, Orp_s, distanceFromWall, relativeDirection, depth, error_flag, soglia_orp, soglia_SOS_parete, soglia_SOS_pos, SOS, Dps_s, alfa, giro, parete_attuale)

    disp("Manovra");
    
    %% Unità di misura 
     
    % Pos_d, Pos_s, soglia_SOS_pos                                                [deg,deg,m]
    % Orp_d, Orp_s, soglia_orp, alfa                                              [rad]
    % relativeDirection                                                           [deg]
    % Dpp_d, Dps_d, Dpp_s, Dps_s, distanceFromWall, depth, soglia_SOS_parete      [m]


    %% Inizializzazione variabili
    
    delta_stato_man = -2 * contatore;
    
    pronti = false;
    
    relativeDirection_rad = deg2rad(relativeDirection);
    
    % Si utilizza la variabile booleana giro, inizializzata nella matlab function "aggiornamento della parete"
    % per determinare il senso di pattugliamento
    if giro == 0 % orario
        inspectionDirection = "clockwise";
    else % antiorario
        inspectionDirection = "counterclockwise";
    end

    %% Preparazione dei riferimenti da fornire si blocchi successivi
          
    Pos_d = [nan; nan; depth];
                                                                            %*****TEST******%
                                                                            %Pos_d = [nan; nan; 0];
    % Distanza dalla parete da mantenere
    Dpp_d = distanceFromWall;
    Dps_d = distanceFromWall;
    
    % Orientazione relativa alla parete
    Orp_d = relativeDirection_rad;
    
    % In questo stato il riferimento di orientazione passato al controllo
    % si riferisce alla parete successiva. Questo rende necessario
    % l'introduzione della variabile "Orp_rif" utilizzata nelle condizioni
    % di switch poiché il valore di stima si riferisce ancora alla parete attuale.
    % I valori alfa corrispondono agli angoli interni ai corner del bacino.
    if (strcmp(inspectionDirection,'clockwise') == 1) % AB-BC-CD-DA
        
        if parete_attuale == 1 % pattugliamento AB, manovra in B
            Orp_rif = relativeDirection_rad + alfa(2); 
        elseif parete_attuale == 2 % pattugliamento BC, manovra in C
            Orp_rif = relativeDirection_rad + alfa(3);
        elseif parete_attuale == 3 % pattugliamento CD, manovra in D
            Orp_rif = relativeDirection_rad + alfa(4);
        else  % pattugliamento DA, manovra in A
            Orp_rif = relativeDirection_rad + alfa(1);
        end
        
    else % AB-DA-CD-BC
        
        if parete_attuale == 1 % pattugliamento AB, manovra in A
            Orp_rif = relativeDirection_rad - alfa(1);
        elseif parete_attuale == 2 % pattugliamento BC, manovra in B
            Orp_rif = relativeDirection_rad - alfa(2);
        elseif parete_attuale == 3 % pattugliamento CD, manovra in C
            Orp_rif = relativeDirection_rad - alfa(3);
        else % pattugliamento DA, manovra in D
            Orp_rif = relativeDirection_rad - alfa(4);
        end
    end
      
    % Transizione di stato effettiva
    delta_current_man = 203 - 202 + contatore;           
    
       
    %% Verifiche
    
    % Verifica di aver mantenuto la corretta profondità e distanza
    % dalle pareti considerate
    if (abs(Pos_s(3) - Pos_d(3)) > soglia_SOS_pos(3) || ...
       abs(Dpp_s - Dpp_d) > soglia_SOS_parete || ...
       abs(Dps_s - Dps_d) > soglia_SOS_parete)
    
        SOS = 1;
        disp("EMERGENZA:");
        
        if (abs(Pos_s(3) - Pos_d(3)) > soglia_SOS_pos(3))
            disp("Rilevato errore sulla profondita");
        end
        if (abs(Dpp_s - Dpp_d) > soglia_SOS_parete)
            disp("Rilevato errore sulla distanza da parete");
        end
        if (abs(Dps_s - Dps_d) > soglia_SOS_parete)
            disp("Rilevato errore sulla distanza da parete successiva");
        end
    end
    
                                                                            %*****TEST******%
                                                                            % if(contatore > 1)
                                                                            %     error_flag = 1;
                                                                            % end

     if error_flag == 1
        disp("EMERGENZA: errore segnalato dagli altri sottosistemi");
        SOS = 1;
     end
     
     
                                                                            %*****TEST******%
                                                                            %Serve per testare di rimanere 
                                                                            %in attesa in questo stato 
                                                                            %test = 0;
                                                                            %if(contatore > 2)%test
                                                                            %    test = 100;
                                                                            %else
                                                                            %    test = 0;
                                                                            %end
                                                                            
    % Si verifica di aver raggiunto l'orientazione desiderata 
    if (SOS == 0 && ...
        abs(Orp_s - Orp_rif) < soglia_orp)    
    
        pronti = true;
        
    end
    
    % La parete viene aggiornata soltanto
    % al termine della fase di manovra incrementando il contatore
    if pronti == true
         contatore = contatore + 1;
    end
    
     
    %% Decisione dello stato successivo
    
    if pronti == true
        if contatore < 4    % Non è ancora il pattugliamento dell'ultima parete 
            
            delta_stato_man = 201 - 203 - 2 * contatore +2;   % Si continua il pattugliamento delle pareti successive  
            
        else    % Completato il pattugliamento dell'ultima parete intera, si esce dal ciclo per
                % effettuare il pattugliamento parziale della parete
                % iniziale che era stata pattugliata solo per metà
                
            delta_stato_man = 204-203 - 2 * contatore +2;         
        end
    end
    
    if SOS == 1
            
            delta_stato_man = 301-203 + - 2 * contatore; %Transizione nello stato di emergenza
    end
        % Si rimane nello stato corrente

end
